simulink subsystem "Motors"  (R2025b)
settings: Solver=VariableStepAuto  StartTime=0.0  StopTime=10.0  RelTol=1e-3
settings Model: Creator=JesseJabezArendse  LastModifiedBy=JesseJabezArendse
settings RTWCC: GPUComputeCapability=3.5

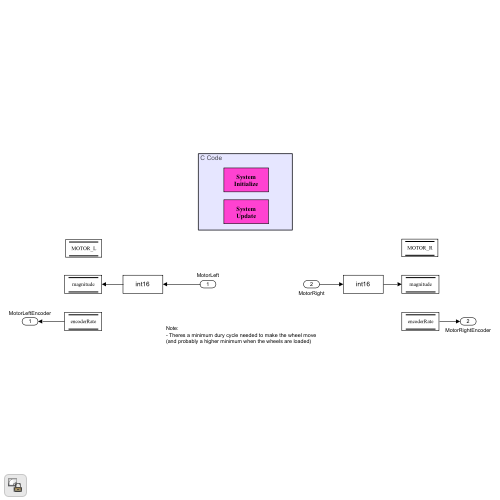
[thumbnail: Simulink's stored preview of the top-level diagram]
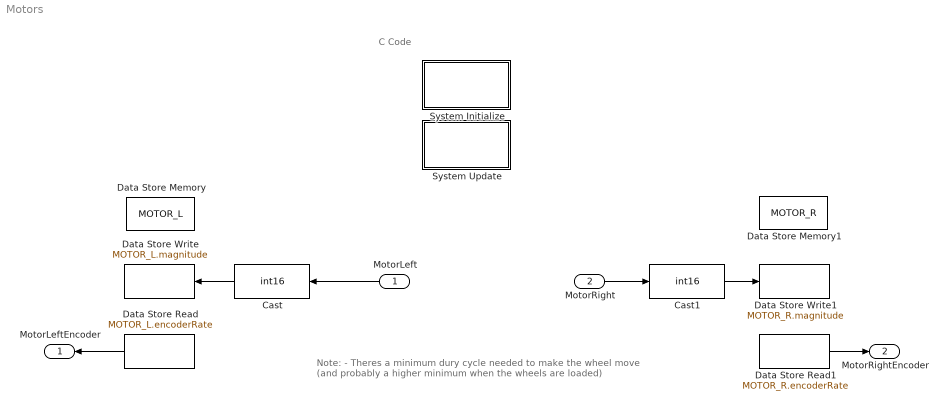
== system Motors ==
  note: Note:
      | - Theres a minimum dury cycle needed to make the wheel move (and probably a higher minimum when the wheels are loaded)
  note: C Code
  MotorLeft : Inport  OutDataTypeStr=int16  PortDimensions=1
  MotorRight : Inport  Port=2  OutDataTypeStr=int16  PortDimensions=1
  Cast : DataTypeConversion  OutDataTypeStr=int16  SaturateOnIntegerOverflow=off  RndMeth=Floor
  Cast1 : DataTypeConversion  OutDataTypeStr=int16  SaturateOnIntegerOverflow=off  RndMeth=Floor
  Data Store Memory : DataStoreMemory  DataStoreName=MOTOR_L  WriteAfterWriteMsg=warning  ShowAdditionalParam=off  OutDataTypeStr=Bus: Motor_t
  Data Store Memory1 : DataStoreMemory  DataStoreName=MOTOR_R  WriteAfterWriteMsg=warning  ShowAdditionalParam=off  OutDataTypeStr=Bus: Motor_t
  Data Store Read : DataStoreRead  DataStoreName=MOTOR_L  DataStoreElements=MOTOR_L.encoderRate  IndexOptions=Index vector (dialog)  Indices=1  OutputSizes=1
  Data Store Read1 : DataStoreRead  DataStoreName=MOTOR_R  DataStoreElements=MOTOR_R.encoderRate  IndexOptions=Index vector (dialog)  Indices=1  OutputSizes=1
  Data Store Write : DataStoreWrite  DataStoreName=MOTOR_L  DataStoreElements=MOTOR_L.magnitude  IndexOptions=Index vector (dialog)  Indices=1  OutputSizes=1
  Data Store Write1 : DataStoreWrite  DataStoreName=MOTOR_R  DataStoreElements=MOTOR_R.magnitude  IndexOptions=Index vector (dialog)  Indices=1  OutputSizes=1
  System Initialize : Subsystem  mask(System Initialize){ShowInLibBrowser=0}
      mask prompts: ShowInLibBrowser "Simulink:masks:CustCodeMaskParam1_MP"
      settings: CopyFcn=cccopyfcn(gcb)  OpenFcn=ccopenfcn('System Initialize Function')
      mask Help: eval('feval(''rtwprivate'',''rtwhelpview'',''rtw_sys_initialize_block'')');
      mask Display: disp('System\nInitialize');
  System Update : Subsystem  mask(System Update){ShowInLibBrowser=0}
      mask prompts: ShowInLibBrowser "Simulink:masks:CustCodeMaskParam1_MP"
      settings: CopyFcn=cccopyfcn(gcb)  OpenFcn=ccopenfcn('System Update Function')
      mask Help: eval('feval(''rtwprivate'',''rtwhelpview'',''rtw_sys_update_block'')');
      mask Display: disp('System\nUpdate');
  MotorLeftEncoder : Outport
  MotorRightEncoder : Outport  Port=2
  wires:
  MotorLeft/1 -> Cast/1
  MotorRight/1 -> Cast1/1
  Data Store Read/1 -> MotorLeftEncoder/1
  Data Store Read1/1 -> MotorRightEncoder/1
  Cast/1 -> Data Store Write/1
  Cast1/1 -> Data Store Write1/1

== system Motors/System Initialize ==

== system Motors/System Update ==
